simulink model "carry_select"  (R2019b)
settings: Solver=VariableStepAuto  StartTime=0.0  StopTime=10.0  RelTol=1e-3
settings Model: Creator=kishan  LastModifiedBy=kishan

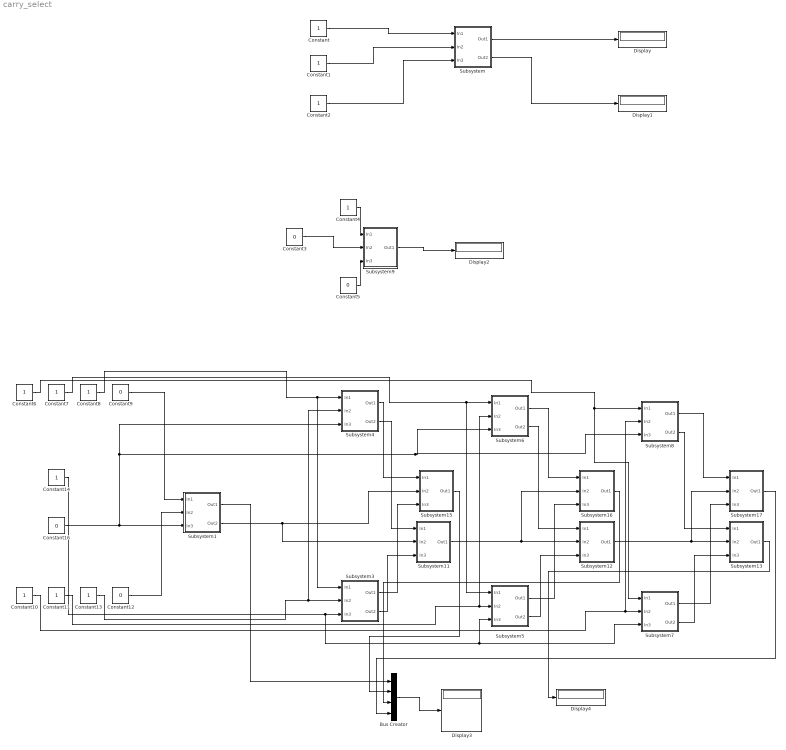
== system carry_select ==
  Bus Creator : BusCreator  Inputs=4
  Constant{,1..2,4,6..8,10..11,13..14} (11 alike) : Constant
  Constant{3,5,9,12,16} (5 alike) : Constant  Value=0
  Display{,1..4} (5 alike) : Display
  Subsystem : Subsystem
  Subsystem1 : Subsystem
  Subsystem11 : Subsystem
  Subsystem12 : Subsystem
  Subsystem13 : Subsystem
  Subsystem15 : Subsystem
  Subsystem16 : Subsystem
  Subsystem17 : Subsystem
  Subsystem3 : Subsystem
  Subsystem4 : Subsystem
  Subsystem5 : Subsystem
  Subsystem6 : Subsystem
  Subsystem7 : Subsystem
  Subsystem8 : Subsystem
  Subsystem9 : Subsystem
  wires:
  Constant/1 -> Subsystem/1(In1)
  Constant1/1 -> Subsystem/2(In2)
  Constant2/1 -> Subsystem/3(In3)
  Subsystem/1(Out1) -> Display/1
  Subsystem/2(Out2) -> Display1/1
  Constant4/1 -> Subsystem9/1(In1)
  Constant3/1 -> Subsystem9/2(In2)
  Constant5/1 -> Subsystem9/3(In3)
  Subsystem9/1(Out1) -> Display2/1
  Constant9/1 -> Subsystem1/1(In1)
  Constant8/1 -> Subsystem3/1(In1), Subsystem4/1(In1)
  Constant7/1 -> Subsystem5/1(In1), Subsystem6/1(In1)
  Constant6/1 -> Subsystem7/1(In1), Subsystem8/1(In1)
  Constant12/1 -> Subsystem1/2(In2)
  Constant13/1 -> Subsystem4/2(In2), Subsystem3/2(In2)
  Constant11/1 -> Subsystem6/2(In2), Subsystem5/2(In2)
  Constant10/1 -> Subsystem8/2(In2), Subsystem7/2(In2)
  Subsystem1/2(Out2) -> Subsystem11/2(In2), Subsystem15/2(In2)
  Subsystem11/1(Out1) -> Subsystem16/2(In2), Subsystem12/2(In2)
  Subsystem12/1(Out1) -> Subsystem17/2(In2), Subsystem13/2(In2)
  Subsystem4/1(Out1) -> Subsystem15/1(In1)
  Subsystem3/1(Out1) -> Subsystem15/3(In3)
  Subsystem4/2(Out2) -> Subsystem11/1(In1)
  Subsystem3/2(Out2) -> Subsystem11/3(In3)
  Subsystem6/1(Out1) -> Subsystem16/1(In1)
  Subsystem5/1(Out1) -> Subsystem16/3(In3)
  Subsystem6/2(Out2) -> Subsystem12/1(In1)
  Subsystem5/2(Out2) -> Subsystem12/3(In3)
  Subsystem8/1(Out1) -> Subsystem17/1(In1)
  Subsystem8/2(Out2) -> Subsystem13/1(In1)
  Subsystem7/1(Out1) -> Subsystem17/3(In3)
  Subsystem7/2(Out2) -> Subsystem13/3(In3)
  Constant16/1 -> Subsystem8/3(In3), Subsystem6/3(In3), Subsystem4/3(In3), Subsystem1/3(In3)
  Constant14/1 -> Subsystem7/3(In3), Subsystem5/3(In3), Subsystem3/3(In3)
  Subsystem1/1(Out1) -> Bus Creator/1
  Subsystem15/1(Out1) -> Bus Creator/2
  Subsystem16/1(Out1) -> Bus Creator/3
  Subsystem17/1(Out1) -> Bus Creator/4
  Bus Creator/1 -> Display3/1
  Subsystem13/1(Out1) -> Display4/1

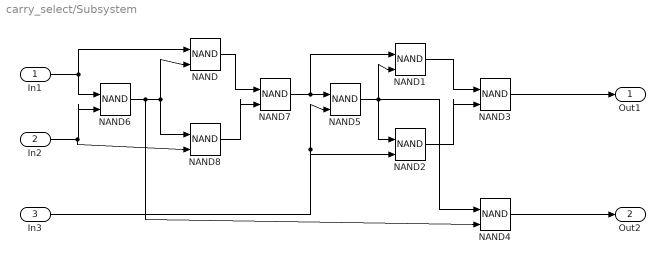
== system carry_select/Subsystem ==
  In1 : Inport
  In2 : Inport  Port=2
  In3 : Inport  Port=3
  NAND{,1..8} (9 alike) : Logic  Operator=NAND  IconShape=distinctive  AllPortsSameDT=off  OutDataTypeStr=boolean
  Out1 : Outport
  Out2 : Outport  Port=2
  wires:
  NAND8/1 -> NAND7/2
  In3/1 -> NAND2/2, NAND5/2
  In1/1 -> NAND6/1, NAND/1
  NAND7/1 -> NAND1/1, NAND5/1
  NAND2/1 -> NAND3/2
  NAND/1 -> NAND7/1
  NAND4/1 -> Out2/1
  NAND1/1 -> NAND3/1
  In2/1 -> NAND8/2, NAND6/2
  NAND6/1 -> NAND4/2, NAND/2, NAND8/1
  NAND3/1 -> Out1/1
  NAND5/1 -> NAND2/1, NAND4/1, NAND1/2

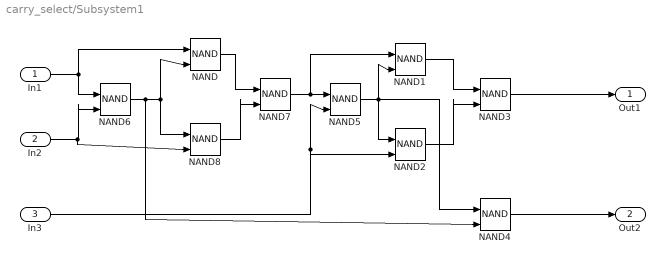
== system carry_select/Subsystem1 ==
  In1 : Inport
  In2 : Inport  Port=2
  In3 : Inport  Port=3
  NAND{,1..8} (9 alike) : Logic  Operator=NAND  IconShape=distinctive  AllPortsSameDT=off  OutDataTypeStr=boolean
  Out1 : Outport
  Out2 : Outport  Port=2
  wires:
  NAND8/1 -> NAND7/2
  In3/1 -> NAND2/2, NAND5/2
  In1/1 -> NAND6/1, NAND/1
  NAND7/1 -> NAND1/1, NAND5/1
  NAND2/1 -> NAND3/2
  NAND/1 -> NAND7/1
  NAND4/1 -> Out2/1
  NAND1/1 -> NAND3/1
  In2/1 -> NAND8/2, NAND6/2
  NAND6/1 -> NAND4/2, NAND/2, NAND8/1
  NAND3/1 -> Out1/1
  NAND5/1 -> NAND2/1, NAND4/1, NAND1/2

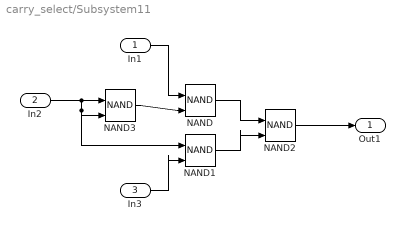
== system carry_select/Subsystem11 ==
  In1 : Inport
  In2 : Inport  Port=2
  In3 : Inport  Port=3
  NAND{,1..3} (4 alike) : Logic  Operator=NAND  IconShape=distinctive  AllPortsSameDT=off  OutDataTypeStr=boolean
  Out1 : Outport
  wires:
  NAND2/1 -> Out1/1
  NAND/1 -> NAND2/1
  In2/1 -> NAND1/1, NAND3/2, NAND3/1
  NAND1/1 -> NAND2/2
  In3/1 -> NAND1/2
  NAND3/1 -> NAND/2
  In1/1 -> NAND/1

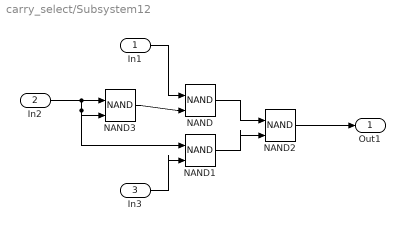
== system carry_select/Subsystem12 ==
  In1 : Inport
  In2 : Inport  Port=2
  In3 : Inport  Port=3
  NAND{,1..3} (4 alike) : Logic  Operator=NAND  IconShape=distinctive  AllPortsSameDT=off  OutDataTypeStr=boolean
  Out1 : Outport
  wires:
  NAND2/1 -> Out1/1
  NAND/1 -> NAND2/1
  In2/1 -> NAND1/1, NAND3/2, NAND3/1
  NAND1/1 -> NAND2/2
  In3/1 -> NAND1/2
  NAND3/1 -> NAND/2
  In1/1 -> NAND/1

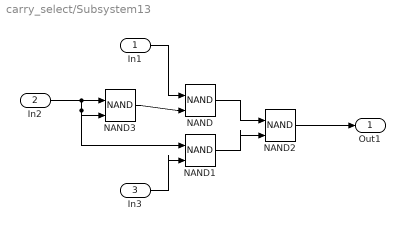
== system carry_select/Subsystem13 ==
  In1 : Inport
  In2 : Inport  Port=2
  In3 : Inport  Port=3
  NAND{,1..3} (4 alike) : Logic  Operator=NAND  IconShape=distinctive  AllPortsSameDT=off  OutDataTypeStr=boolean
  Out1 : Outport
  wires:
  NAND2/1 -> Out1/1
  NAND/1 -> NAND2/1
  In2/1 -> NAND1/1, NAND3/2, NAND3/1
  NAND1/1 -> NAND2/2
  In3/1 -> NAND1/2
  NAND3/1 -> NAND/2
  In1/1 -> NAND/1

== system carry_select/Subsystem15 ==
  In1 : Inport
  In2 : Inport  Port=2
  In3 : Inport  Port=3
  NAND{,1..3} (4 alike) : Logic  Operator=NAND  IconShape=distinctive  AllPortsSameDT=off  OutDataTypeStr=boolean
  Out1 : Outport
  wires:
  NAND2/1 -> Out1/1
  NAND/1 -> NAND2/1
  In2/1 -> NAND1/1, NAND3/2, NAND3/1
  NAND1/1 -> NAND2/2
  In3/1 -> NAND1/2
  NAND3/1 -> NAND/2
  In1/1 -> NAND/1

== system carry_select/Subsystem16 ==
  In1 : Inport
  In2 : Inport  Port=2
  In3 : Inport  Port=3
  NAND{,1..3} (4 alike) : Logic  Operator=NAND  IconShape=distinctive  AllPortsSameDT=off  OutDataTypeStr=boolean
  Out1 : Outport
  wires:
  NAND2/1 -> Out1/1
  NAND/1 -> NAND2/1
  In2/1 -> NAND1/1, NAND3/2, NAND3/1
  NAND1/1 -> NAND2/2
  In3/1 -> NAND1/2
  NAND3/1 -> NAND/2
  In1/1 -> NAND/1

== system carry_select/Subsystem17 ==
  In1 : Inport
  In2 : Inport  Port=2
  In3 : Inport  Port=3
  NAND{,1..3} (4 alike) : Logic  Operator=NAND  IconShape=distinctive  AllPortsSameDT=off  OutDataTypeStr=boolean
  Out1 : Outport
  wires:
  NAND2/1 -> Out1/1
  NAND/1 -> NAND2/1
  In2/1 -> NAND1/1, NAND3/2, NAND3/1
  NAND1/1 -> NAND2/2
  In3/1 -> NAND1/2
  NAND3/1 -> NAND/2
  In1/1 -> NAND/1

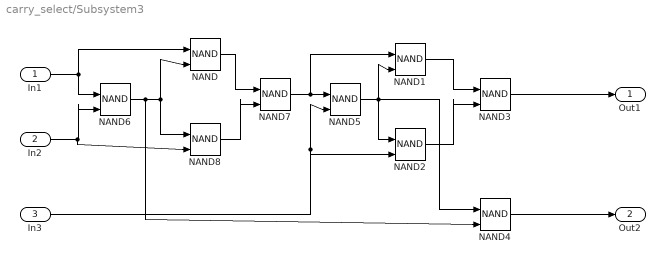
== system carry_select/Subsystem3 ==
  In1 : Inport
  In2 : Inport  Port=2
  In3 : Inport  Port=3
  NAND{,1..8} (9 alike) : Logic  Operator=NAND  IconShape=distinctive  AllPortsSameDT=off  OutDataTypeStr=boolean
  Out1 : Outport
  Out2 : Outport  Port=2
  wires:
  NAND8/1 -> NAND7/2
  In3/1 -> NAND2/2, NAND5/2
  In1/1 -> NAND6/1, NAND/1
  NAND7/1 -> NAND1/1, NAND5/1
  NAND2/1 -> NAND3/2
  NAND/1 -> NAND7/1
  NAND4/1 -> Out2/1
  NAND1/1 -> NAND3/1
  In2/1 -> NAND8/2, NAND6/2
  NAND6/1 -> NAND4/2, NAND/2, NAND8/1
  NAND3/1 -> Out1/1
  NAND5/1 -> NAND2/1, NAND4/1, NAND1/2

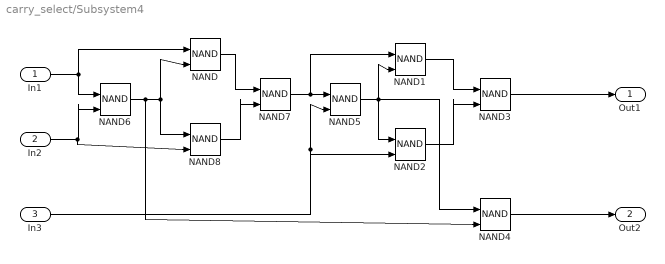
== system carry_select/Subsystem4 ==
  In1 : Inport
  In2 : Inport  Port=2
  In3 : Inport  Port=3
  NAND{,1..8} (9 alike) : Logic  Operator=NAND  IconShape=distinctive  AllPortsSameDT=off  OutDataTypeStr=boolean
  Out1 : Outport
  Out2 : Outport  Port=2
  wires:
  NAND8/1 -> NAND7/2
  In3/1 -> NAND2/2, NAND5/2
  In1/1 -> NAND6/1, NAND/1
  NAND7/1 -> NAND1/1, NAND5/1
  NAND2/1 -> NAND3/2
  NAND/1 -> NAND7/1
  NAND4/1 -> Out2/1
  NAND1/1 -> NAND3/1
  In2/1 -> NAND8/2, NAND6/2
  NAND6/1 -> NAND4/2, NAND/2, NAND8/1
  NAND3/1 -> Out1/1
  NAND5/1 -> NAND2/1, NAND4/1, NAND1/2

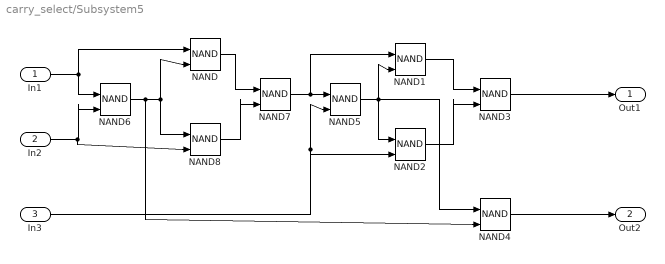
== system carry_select/Subsystem5 ==
  In1 : Inport
  In2 : Inport  Port=2
  In3 : Inport  Port=3
  NAND{,1..8} (9 alike) : Logic  Operator=NAND  IconShape=distinctive  AllPortsSameDT=off  OutDataTypeStr=boolean
  Out1 : Outport
  Out2 : Outport  Port=2
  wires:
  NAND8/1 -> NAND7/2
  In3/1 -> NAND2/2, NAND5/2
  In1/1 -> NAND6/1, NAND/1
  NAND7/1 -> NAND1/1, NAND5/1
  NAND2/1 -> NAND3/2
  NAND/1 -> NAND7/1
  NAND4/1 -> Out2/1
  NAND1/1 -> NAND3/1
  In2/1 -> NAND8/2, NAND6/2
  NAND6/1 -> NAND4/2, NAND/2, NAND8/1
  NAND3/1 -> Out1/1
  NAND5/1 -> NAND2/1, NAND4/1, NAND1/2

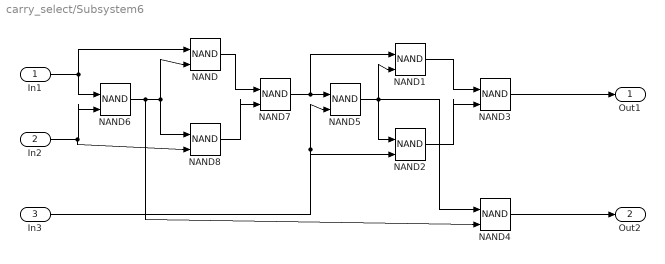
== system carry_select/Subsystem6 ==
  In1 : Inport
  In2 : Inport  Port=2
  In3 : Inport  Port=3
  NAND{,1..8} (9 alike) : Logic  Operator=NAND  IconShape=distinctive  AllPortsSameDT=off  OutDataTypeStr=boolean
  Out1 : Outport
  Out2 : Outport  Port=2
  wires:
  NAND8/1 -> NAND7/2
  In3/1 -> NAND2/2, NAND5/2
  In1/1 -> NAND6/1, NAND/1
  NAND7/1 -> NAND1/1, NAND5/1
  NAND2/1 -> NAND3/2
  NAND/1 -> NAND7/1
  NAND4/1 -> Out2/1
  NAND1/1 -> NAND3/1
  In2/1 -> NAND8/2, NAND6/2
  NAND6/1 -> NAND4/2, NAND/2, NAND8/1
  NAND3/1 -> Out1/1
  NAND5/1 -> NAND2/1, NAND4/1, NAND1/2

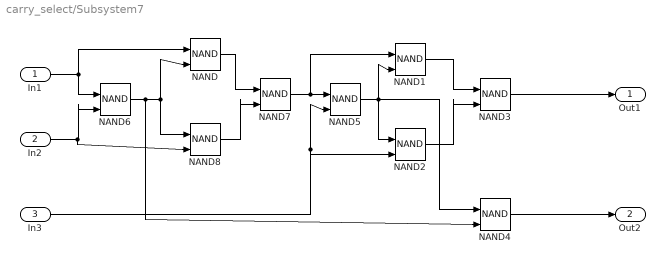
== system carry_select/Subsystem7 ==
  In1 : Inport
  In2 : Inport  Port=2
  In3 : Inport  Port=3
  NAND{,1..8} (9 alike) : Logic  Operator=NAND  IconShape=distinctive  AllPortsSameDT=off  OutDataTypeStr=boolean
  Out1 : Outport
  Out2 : Outport  Port=2
  wires:
  NAND8/1 -> NAND7/2
  In3/1 -> NAND2/2, NAND5/2
  In1/1 -> NAND6/1, NAND/1
  NAND7/1 -> NAND1/1, NAND5/1
  NAND2/1 -> NAND3/2
  NAND/1 -> NAND7/1
  NAND4/1 -> Out2/1
  NAND1/1 -> NAND3/1
  In2/1 -> NAND8/2, NAND6/2
  NAND6/1 -> NAND4/2, NAND/2, NAND8/1
  NAND3/1 -> Out1/1
  NAND5/1 -> NAND2/1, NAND4/1, NAND1/2

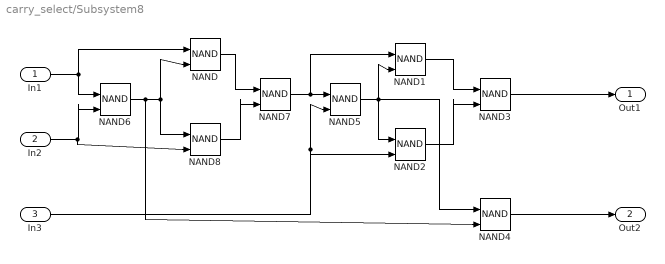
== system carry_select/Subsystem8 ==
  In1 : Inport
  In2 : Inport  Port=2
  In3 : Inport  Port=3
  NAND{,1..8} (9 alike) : Logic  Operator=NAND  IconShape=distinctive  AllPortsSameDT=off  OutDataTypeStr=boolean
  Out1 : Outport
  Out2 : Outport  Port=2
  wires:
  NAND8/1 -> NAND7/2
  In3/1 -> NAND2/2, NAND5/2
  In1/1 -> NAND6/1, NAND/1
  NAND7/1 -> NAND1/1, NAND5/1
  NAND2/1 -> NAND3/2
  NAND/1 -> NAND7/1
  NAND4/1 -> Out2/1
  NAND1/1 -> NAND3/1
  In2/1 -> NAND8/2, NAND6/2
  NAND6/1 -> NAND4/2, NAND/2, NAND8/1
  NAND3/1 -> Out1/1
  NAND5/1 -> NAND2/1, NAND4/1, NAND1/2

== system carry_select/Subsystem9 ==
  In1 : Inport
  In2 : Inport  Port=2
  In3 : Inport  Port=3
  NAND{,1..3} (4 alike) : Logic  Operator=NAND  IconShape=distinctive  AllPortsSameDT=off  OutDataTypeStr=boolean
  Out1 : Outport
  wires:
  NAND2/1 -> Out1/1
  NAND/1 -> NAND2/1
  In2/1 -> NAND1/1, NAND3/2, NAND3/1
  NAND1/1 -> NAND2/2
  In3/1 -> NAND1/2
  NAND3/1 -> NAND/2
  In1/1 -> NAND/1
